simulink library "kalmanlib"  (Simulink 7.0)
undefined symbols (not defined in the file): dt, P0, Q, seed1, tS, x0
libraries: kalmanlib x10, simulink x6
(part 2 of 2)

== system kalmanlib/kalman filter/Extended Kalman Filter (System)/P corrector ==
  K : Inport  OutDataType=sfix(16)  OutScaling=2^0
  Pk' : Inport  Port=2  OutDataType=sfix(16)  OutScaling=2^0
  Add1 : Sum  Inputs=+-  OutDataType=sfix(16)  OutScaling=2^-10
  Eins : Constant  Value=eye(size(P0))  VectorParams1D=off  OutDataType=sfix(16)  OutScaling=2^0
  Gain1 : Gain  Gain=H  Multiplication=Matrix(u*K)  ParameterDataType=sfix(16)  ParameterScaling=2^0  OutDataType=sfix(16)  OutScaling=2^0
  Product1 : Product  Multiplication=Matrix(*)  OutDataType=sfix(16)  OutScaling=2^0  RndMeth=Zero
  Pk : Outport  OutDataType=sfix(16)  OutScaling=2^0
  wires:
  Product1/1 -> Pk/1
  Pk'/1 -> Product1/2
  Gain1/1 -> Add1/2
  Eins/1 -> Add1/1
  Add1/1 -> Product1/1
  K/1 -> Gain1/1

== system kalmanlib/kalman filter/Extended Kalman Filter (System)/P predictor ==
  Pk : Inport  OutDataType=sfix(16)  OutScaling=2^0
  A : Inport  Port=2  OutDataType=sfix(16)  OutScaling=2^0
  Add : Sum  OutDataType=sfix(16)  OutScaling=2^-10
  Math Function : Math  Operator=transpose  OutDataType=sfix(16)  OutScaling=2^0  SaturateOnIntegerOverflow=on
  Product : Product  Inputs=3  Multiplication=Matrix(*)  OutDataType=sfix(16)  OutScaling=2^0  RndMeth=Zero
  Q : Constant  Value=Q  VectorParams1D=off  OutDataType=sfix(16)  OutScaling=2^0
  Pk' : Outport  OutDataType=sfix(16)  OutScaling=2^0
  wires:
  A/1 -> Math Function/1, Product/1
  Pk/1 -> Product/2
  Math Function/1 -> Product/3
  Product/1 -> Add/1
  Q/1 -> Add/2
  Add/1 -> Pk'/1

== system kalmanlib/kalman filter/Extended Kalman Filter (System)/System (lin) ==
  note: Trivial System
      | y = x
  x : Inport  OutDataType=sfix(16)  OutScaling=2^0
  One : MATLABFcn  MATLABFcn=eye(size(u,1))  Output1D=off
  f(x) : Outport  OutDataType=sfix(16)  OutScaling=2^0
  A : Outport  Port=2  OutDataType=sfix(16)  OutScaling=2^0
  wires:
  x/1 -> One/1, f(x)/1
  One/1 -> A/1

== system kalmanlib/kalman filter/Extended Kalman Filter (System)/x corrector ==
  xk' : Inport  OutDataType=sfix(16)  OutScaling=2^0
  zk : Inport  Port=2  OutDataType=sfix(16)  OutScaling=2^0
  K : Inport  Port=3  OutDataType=sfix(16)  OutScaling=2^0
  Add : Sum  OutDataType=sfix(16)  OutScaling=2^-10
  Add1 : Sum  Inputs=-+  OutDataType=sfix(16)  OutScaling=2^-10
  Gain1 : Gain  Gain=H  Multiplication=Matrix(K*u)  ParameterDataType=sfix(16)  ParameterScaling=2^0  OutDataType=sfix(16)  OutScaling=2^0
  Product1 : Product  Multiplication=Matrix(*)  OutDataType=sfix(16)  OutScaling=2^0  RndMeth=Zero
  x(k+1) : Outport  OutDataType=sfix(16)  OutScaling=2^0
  wires:
  Gain1/1 -> Add1/1
  Add/1 -> x(k+1)/1
  xk'/1 -> Gain1/1, Add/1
  Product1/1 -> Add/2
  K/1 -> Product1/1
  zk/1 -> Add1/2
  Add1/1 -> Product1/2

== system kalmanlib/kalman filter/Extended Kalman Filter (System)/x predictor ==
  f(xk) : Inport  OutDataType=sfix(16)  OutScaling=2^0
  uk : Inport  Port=2  OutDataType=sfix(16)  OutScaling=2^0
  Add : Sum  OutDataType=sfix(16)  OutScaling=2^-10
  Gain1 : Gain  Gain=B  Multiplication=Matrix(K*u)  ParameterDataType=sfix(16)  ParameterScaling=2^0  OutDataType=sfix(16)  OutScaling=2^0
  x(k+1)' : Outport  OutDataType=sfix(16)  OutScaling=2^0
  wires:
  Add/1 -> x(k+1)'/1
  Gain1/1 -> Add/2
  uk/1 -> Gain1/1
  f(xk)/1 -> Add/1

== system kalmanlib/kalman filter/Kalman Filter/K corrector ==
  Pk' : Inport  OutDataType=sfix(16)  OutScaling=2^0
  Add : Sum  OutDataType=sfix(16)  OutScaling=2^-10
  C : Constant  Value=H  VectorParams1D=off  OutDataType=sfix(16)  OutScaling=2^0
  C' : Constant  Value=H'  VectorParams1D=off  OutDataType=sfix(16)  OutScaling=2^0
  Product : Product  Inputs=3  Multiplication=Matrix(*)  OutDataType=sfix(16)  OutScaling=2^0  RndMeth=Zero
  Product1 : Product  Inputs=**/  Multiplication=Matrix(*)  OutDataType=sfix(16)  OutScaling=2^0  RndMeth=Zero
  R : Constant  Value=R  OutDataType=sfix(16)  OutScaling=2^0
  K : Outport  OutDataType=sfix(16)  OutScaling=2^0
  wires:
  C'/1 -> Product/3, Product1/2
  R/1 -> Add/2
  Product/1 -> Add/1
  Pk'/1 -> Product/2, Product1/1
  C/1 -> Product/1
  Product1/1 -> K/1
  Add/1 -> Product1/3

== system kalmanlib/kalman filter/Kalman Filter/P corrector ==
  K : Inport  OutDataType=sfix(16)  OutScaling=2^0
  Pk' : Inport  Port=2  OutDataType=sfix(16)  OutScaling=2^0
  Add1 : Sum  Inputs=+-  OutDataType=sfix(16)  OutScaling=2^-10
  Eins : Constant  Value=eye(size(P0))  VectorParams1D=off  OutDataType=sfix(16)  OutScaling=2^0
  Gain1 : Gain  Gain=H  Multiplication=Matrix(u*K)  ParameterDataType=sfix(16)  ParameterScaling=2^0  OutDataType=sfix(16)  OutScaling=2^0
  Product1 : Product  Multiplication=Matrix(*)  OutDataType=sfix(16)  OutScaling=2^0  RndMeth=Zero
  Pk : Outport  OutDataType=sfix(16)  OutScaling=2^0
  wires:
  Product1/1 -> Pk/1
  Pk'/1 -> Product1/2
  Gain1/1 -> Add1/2
  Eins/1 -> Add1/1
  Add1/1 -> Product1/1
  K/1 -> Gain1/1

== system kalmanlib/kalman filter/Kalman Filter/P predictor ==
  Pk : Inport  OutDataType=sfix(16)  OutScaling=2^0
  A : Constant  Value=A  OutDataType=sfix(16)  OutScaling=2^0
  A' : Constant  Value=A'  OutDataType=sfix(16)  OutScaling=2^0
  Add : Sum  OutDataType=sfix(16)  OutScaling=2^-10
  Product : Product  Inputs=3  Multiplication=Matrix(*)  OutDataType=sfix(16)  OutScaling=2^0  RndMeth=Zero
  Q : Constant  Value=Q  VectorParams1D=off  OutDataType=sfix(16)  OutScaling=2^0
  Pk' : Outport  OutDataType=sfix(16)  OutScaling=2^0
  wires:
  A/1 -> Product/1
  Pk/1 -> Product/2
  A'/1 -> Product/3
  Product/1 -> Add/1
  Q/1 -> Add/2
  Add/1 -> Pk'/1

== system kalmanlib/kalman filter/Kalman Filter/x corrector ==
  xk' : Inport  OutDataType=sfix(16)  OutScaling=2^0
  zk : Inport  Port=2  OutDataType=sfix(16)  OutScaling=2^0
  K : Inport  Port=3  OutDataType=sfix(16)  OutScaling=2^0
  Add : Sum  OutDataType=sfix(16)  OutScaling=2^-10
  Add1 : Sum  Inputs=-+  OutDataType=sfix(16)  OutScaling=2^-10
  Gain1 : Gain  Gain=H  Multiplication=Matrix(K*u)  ParameterDataType=sfix(16)  ParameterScaling=2^0  OutDataType=sfix(16)  OutScaling=2^0
  Product1 : Product  Multiplication=Matrix(*)  OutDataType=sfix(16)  OutScaling=2^0  RndMeth=Zero
  x(k+1) : Outport  OutDataType=sfix(16)  OutScaling=2^0
  wires:
  Gain1/1 -> Add1/1
  Add/1 -> x(k+1)/1
  xk'/1 -> Gain1/1, Add/1
  Product1/1 -> Add/2
  K/1 -> Product1/1
  zk/1 -> Add1/2
  Add1/1 -> Product1/2

== system kalmanlib/kalman filter/Kalman Filter/x predictor ==
  xk : Inport  OutDataType=sfix(16)  OutScaling=2^0
  uk : Inport  Port=2  OutDataType=sfix(16)  OutScaling=2^0
  Add : Sum  OutDataType=sfix(16)  OutScaling=2^-10
  Gain : Gain  Gain=A  Multiplication=Matrix(K*u)  ParameterDataType=sfix(16)  ParameterScaling=2^0  OutDataType=sfix(16)  OutScaling=2^0
  Gain1 : Gain  Gain=B  Multiplication=Matrix(K*u)  ParameterDataType=sfix(16)  ParameterScaling=2^0  OutDataType=sfix(16)  OutScaling=2^0
  x(k+1)' : Outport  OutDataType=sfix(16)  OutScaling=2^0
  wires:
  Add/1 -> x(k+1)'/1
  Gain1/1 -> Add/2
  Gain/1 -> Add/1
  uk/1 -> Gain1/1
  xk/1 -> Gain/1

== system kalmanlib/kalman filter/Kalman Filter A(t), Q(t), B(t) H(t), R(t)/K corrector ==
  Pk' : Inport  OutDataType=sfix(16)  OutScaling=2^0
  H : Inport  Port=2  OutDataType=sfix(16)  OutScaling=2^0
  R : Inport  Port=3  OutDataType=sfix(16)  OutScaling=2^0
  Add : Sum  OutDataType=sfix(16)  OutScaling=2^-10
  Math Function : Math  Operator=transpose  OutDataType=sfix(16)  OutScaling=2^0  SaturateOnIntegerOverflow=on
  Product : Product  Inputs=3  Multiplication=Matrix(*)  OutDataType=sfix(16)  OutScaling=2^0  RndMeth=Zero
  Product1 : Product  Inputs=**/  Multiplication=Matrix(*)  OutDataType=sfix(16)  OutScaling=2^0  RndMeth=Zero
  K : Outport  OutDataType=sfix(16)  OutScaling=2^0
  wires:
  R/1 -> Add/2
  Product/1 -> Add/1
  Math Function/1 -> Product/3, Product1/2
  Pk'/1 -> Product/2, Product1/1
  H/1 -> Product/1, Math Function/1
  Product1/1 -> K/1
  Add/1 -> Product1/3

== system kalmanlib/kalman filter/Kalman Filter A(t), Q(t), B(t) H(t), R(t)/P corrector ==
  K : Inport  OutDataType=sfix(16)  OutScaling=2^0
  Pk' : Inport  Port=2  OutDataType=sfix(16)  OutScaling=2^0
  H : Inport  Port=3  OutDataType=sfix(16)  OutScaling=2^0
  Add1 : Sum  Inputs=+-  OutDataType=sfix(16)  OutScaling=2^-10
  Eins : Constant  Value=eye(size(P0))  VectorParams1D=off  OutDataType=sfix(16)  OutScaling=2^0
  Product1 : Product  Multiplication=Matrix(*)  OutDataType=sfix(16)  OutScaling=2^0  RndMeth=Zero
  Product2 : Product  Multiplication=Matrix(*)  OutDataType=sfix(16)  OutScaling=2^0  RndMeth=Zero
  Pk : Outport  OutDataType=sfix(16)  OutScaling=2^0
  wires:
  Product1/1 -> Pk/1
  Pk'/1 -> Product1/2
  Product2/1 -> Add1/2
  Eins/1 -> Add1/1
  Add1/1 -> Product1/1
  K/1 -> Product2/1
  H/1 -> Product2/2

== system kalmanlib/kalman filter/Kalman Filter A(t), Q(t), B(t) H(t), R(t)/P predictor ==
  Pk : Inport  OutDataType=sfix(16)  OutScaling=2^0
  A : Inport  Port=2  OutDataType=sfix(16)  OutScaling=2^0
  Q : Inport  Port=3  OutDataType=sfix(16)  OutScaling=2^0
  Add : Sum  OutDataType=sfix(16)  OutScaling=2^-10
  Math Function : Math  Operator=transpose  OutDataType=sfix(16)  OutScaling=2^0  SaturateOnIntegerOverflow=on
  Product : Product  Inputs=3  Multiplication=Matrix(*)  OutDataType=sfix(16)  OutScaling=2^0  RndMeth=Zero
  Pk' : Outport  OutDataType=sfix(16)  OutScaling=2^0
  wires:
  Q/1 -> Add/2
  A/1 -> Math Function/1, Product/1
  Pk/1 -> Product/2
  Math Function/1 -> Product/3
  Product/1 -> Add/1
  Add/1 -> Pk'/1

== system kalmanlib/kalman filter/Kalman Filter A(t), Q(t), B(t) H(t), R(t)/x corrector ==
  xk' : Inport  OutDataType=sfix(16)  OutScaling=2^0
  zk : Inport  Port=2  OutDataType=sfix(16)  OutScaling=2^0
  K : Inport  Port=3  OutDataType=sfix(16)  OutScaling=2^0
  h(xk') : Inport  Port=4  OutDataType=sfix(16)  OutScaling=2^0
  Add : Sum  OutDataType=sfix(16)  OutScaling=2^-10
  Add1 : Sum  Inputs=-+  OutDataType=sfix(16)  OutScaling=2^-10
  Product1 : Product  Multiplication=Matrix(*)  OutDataType=sfix(16)  OutScaling=2^0  RndMeth=Zero
  x(k+1) : Outport  OutDataType=sfix(16)  OutScaling=2^0
  wires:
  Add/1 -> x(k+1)/1
  xk'/1 -> Add/1
  Product1/1 -> Add/2
  K/1 -> Product1/1
  zk/1 -> Add1/2
  Add1/1 -> Product1/2
  h(xk')/1 -> Add1/1

== system kalmanlib/kalman filter/Kalman Filter A(t), Q(t), B(t) H(t), R(t)/x predictor ==
  xk : Inport  OutDataType=sfix(16)  OutScaling=2^0
  uk : Inport  Port=2  OutDataType=sfix(16)  OutScaling=2^0
  A : Inport  Port=3  OutDataType=sfix(16)  OutScaling=2^0
  B : Inport  Port=4  OutDataType=sfix(16)  OutScaling=2^0
  Add : Sum  OutDataType=sfix(16)  OutScaling=2^-10
  Product1 : Product  Multiplication=Matrix(*)  OutDataType=sfix(16)  OutScaling=2^0  RndMeth=Zero
  Product2 : Product  Multiplication=Matrix(*)  OutDataType=sfix(16)  OutScaling=2^0  RndMeth=Zero
  x(k+1)' : Outport  OutDataType=sfix(16)  OutScaling=2^0
  wires:
  B/1 -> Product1/1
  A/1 -> Product2/1
  Add/1 -> x(k+1)'/1
  Product1/1 -> Add/2
  Product2/1 -> Add/1
  uk/1 -> Product1/2
  xk/1 -> Product2/2

== system kalmanlib/kalman filter/Kalman Filter H(t), R(t)/K corrector ==
  Pk' : Inport  OutDataType=sfix(16)  OutScaling=2^0
  H : Inport  Port=2  OutDataType=sfix(16)  OutScaling=2^0
  R : Inport  Port=3  OutDataType=sfix(16)  OutScaling=2^0
  Add : Sum  OutDataType=sfix(16)  OutScaling=2^-10
  Math Function : Math  Operator=transpose  OutDataType=sfix(16)  OutScaling=2^0  SaturateOnIntegerOverflow=on
  Product : Product  Inputs=3  Multiplication=Matrix(*)  OutDataType=sfix(16)  OutScaling=2^0  RndMeth=Zero
  Product1 : Product  Inputs=**/  Multiplication=Matrix(*)  OutDataType=sfix(16)  OutScaling=2^0  RndMeth=Zero
  K : Outport  OutDataType=sfix(16)  OutScaling=2^0
  wires:
  Add/1 -> Product1/3
  Product1/1 -> K/1
  H/1 -> Math Function/1, Product/1
  Pk'/1 -> Product1/1, Product/2
  Math Function/1 -> Product1/2, Product/3
  Product/1 -> Add/1
  R/1 -> Add/2

== system kalmanlib/kalman filter/Kalman Filter H(t), R(t)/P corrector ==
  K : Inport  OutDataType=sfix(16)  OutScaling=2^0
  Pk' : Inport  Port=2  OutDataType=sfix(16)  OutScaling=2^0
  H : Inport  Port=3  OutDataType=sfix(16)  OutScaling=2^0
  Add1 : Sum  Inputs=+-  OutDataType=sfix(16)  OutScaling=2^-10
  Eins : Constant  Value=eye(size(P0))  VectorParams1D=off  OutDataType=sfix(16)  OutScaling=2^0
  Product1 : Product  Multiplication=Matrix(*)  OutDataType=sfix(16)  OutScaling=2^0  RndMeth=Zero
  Product2 : Product  Multiplication=Matrix(*)  OutDataType=sfix(16)  OutScaling=2^0  RndMeth=Zero
  Pk : Outport  OutDataType=sfix(16)  OutScaling=2^0
  wires:
  H/1 -> Product2/2
  K/1 -> Product2/1
  Add1/1 -> Product1/1
  Eins/1 -> Add1/1
  Product2/1 -> Add1/2
  Pk'/1 -> Product1/2
  Product1/1 -> Pk/1

== system kalmanlib/kalman filter/Kalman Filter H(t), R(t)/P predictor ==
  Pk : Inport  OutDataType=sfix(16)  OutScaling=2^0
  A : Constant  Value=A  OutDataType=sfix(16)  OutScaling=2^0
  A' : Constant  Value=A'  OutDataType=sfix(16)  OutScaling=2^0
  Add : Sum  OutDataType=sfix(16)  OutScaling=2^-10
  Product : Product  Inputs=3  Multiplication=Matrix(*)  OutDataType=sfix(16)  OutScaling=2^0  RndMeth=Zero
  Q : Constant  Value=Q  VectorParams1D=off  OutDataType=sfix(16)  OutScaling=2^0
  Pk' : Outport  OutDataType=sfix(16)  OutScaling=2^0
  wires:
  Add/1 -> Pk'/1
  Q/1 -> Add/2
  Product/1 -> Add/1
  A'/1 -> Product/3
  Pk/1 -> Product/2
  A/1 -> Product/1

== system kalmanlib/kalman filter/Kalman Filter H(t), R(t)/x corrector ==
  xk' : Inport  OutDataType=sfix(16)  OutScaling=2^0
  zk : Inport  Port=2  OutDataType=sfix(16)  OutScaling=2^0
  K : Inport  Port=3  OutDataType=sfix(16)  OutScaling=2^0
  h(xk') : Inport  Port=4  OutDataType=sfix(16)  OutScaling=2^0
  Add : Sum  OutDataType=sfix(16)  OutScaling=2^-10
  Add1 : Sum  Inputs=-+  OutDataType=sfix(16)  OutScaling=2^-10
  Product1 : Product  Multiplication=Matrix(*)  OutDataType=sfix(16)  OutScaling=2^0  RndMeth=Zero
  x(k+1) : Outport  OutDataType=sfix(16)  OutScaling=2^0
  wires:
  h(xk')/1 -> Add1/1
  Add1/1 -> Product1/2
  zk/1 -> Add1/2
  K/1 -> Product1/1
  Product1/1 -> Add/2
  xk'/1 -> Add/1
  Add/1 -> x(k+1)/1

== system kalmanlib/kalman filter/Kalman Filter H(t), R(t)/x predictor ==
  xk : Inport  OutDataType=sfix(16)  OutScaling=2^0
  uk : Inport  Port=2  OutDataType=sfix(16)  OutScaling=2^0
  Add : Sum  OutDataType=sfix(16)  OutScaling=2^-10
  Gain : Gain  Gain=A  Multiplication=Matrix(K*u)  ParameterDataType=sfix(16)  ParameterScaling=2^0  OutDataType=sfix(16)  OutScaling=2^0
  Gain1 : Gain  Gain=B  Multiplication=Matrix(K*u)  ParameterDataType=sfix(16)  ParameterScaling=2^0  OutDataType=sfix(16)  OutScaling=2^0
  x(k+1)' : Outport  OutDataType=sfix(16)  OutScaling=2^0
  wires:
  xk/1 -> Gain/1
  uk/1 -> Gain1/1
  Gain/1 -> Add/1
  Gain1/1 -> Add/2
  Add/1 -> x(k+1)'/1

== system kalmanlib/models/Two-Phase Measurement/Hit Test ==
  Digital Clock : DigitalClock  SampleTime=dt
  Gain : Gain  Gain=1/(n*dt)  ParameterDataType=sfix(16)  ParameterScaling=2^0  OutDataType=sfix(16)  OutScaling=2^0
  Gain1 : Gain  Gain=n*dt  ParameterDataType=sfix(16)  ParameterScaling=2^0  OutDataType=sfix(16)  OutScaling=2^0
  Interval Test : simulink/Logic and Bit Operations/Interval Test  SystemSampleTime=-1  IntervalClosedRight=on  uplimit=100*eps  IntervalClosedLeft=on  lowlimit=-100*eps  LogicOutDataTypeMode=boolean
  Rounding Function : Rounding
  Subtract : Sum  Inputs=+-  OutDataType=sfix(16)  OutScaling=2^-10
  hit : Outport  OutDataType=sfix(16)  OutScaling=2^0
  wires:
  Digital Clock/1 -> Gain/1, Subtract/1
  Gain/1 -> Rounding Function/1
  Rounding Function/1 -> Gain1/1
  Gain1/1 -> Subtract/2
  Subtract/1 -> Interval Test/1
  Interval Test/1 -> hit/1
